simulink model "lead_increasing_space_gap"  (R2025a)
settings: Solver=VariableStepAuto  StartTime=0.0  StopTime=20  RelTol=1e-3
settings Model: Creator=sanborkl  LastModifiedBy=sanborkl

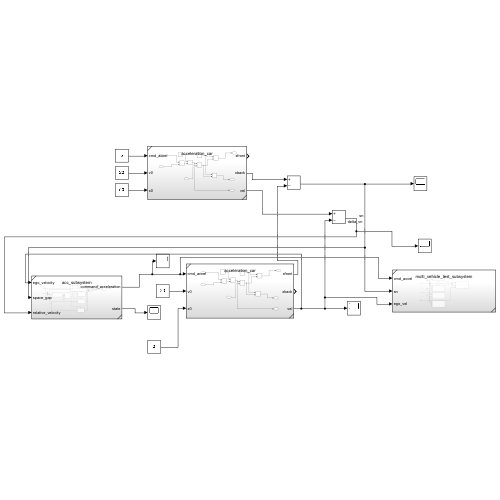
[thumbnail: Simulink's stored preview of the top-level diagram]
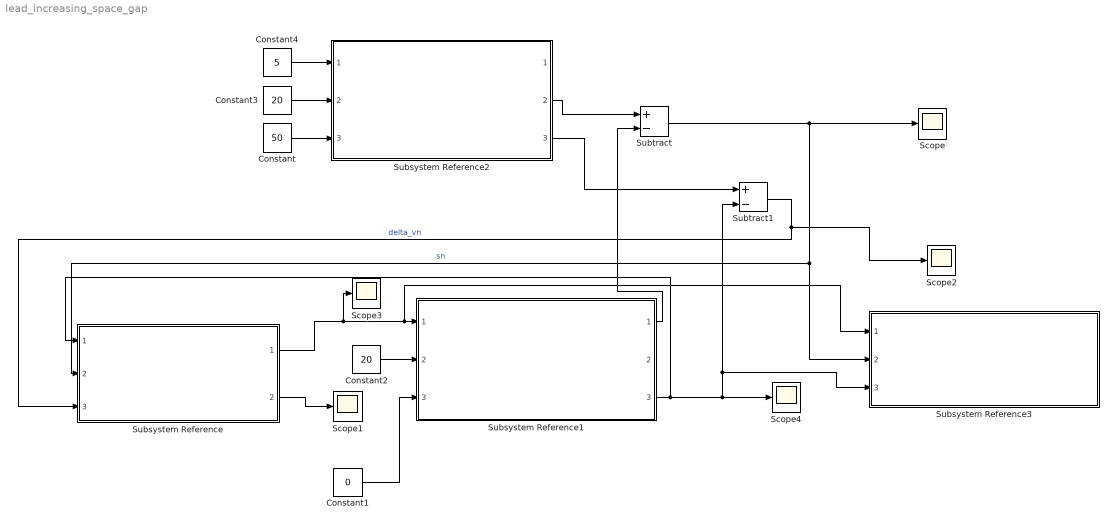
== system lead_increasing_space_gap ==
  Constant : Constant  Value=50
  Constant1 : Constant  Value=0
  Constant2 : Constant  Value=20
  Constant3 : Constant  Value=20
  Constant4 : Constant  Value=5
  Scope{,1..4} (5 alike) : Scope
      Scope settings: ActiveDisplayYMinimum=7.0577298305674168  ActiveDisplayYMaximum=50.060252241048069
      Scope1 settings: ActiveDisplayYMinimum=-1  ActiveDisplayYMaximum=1  DataLoggingVariableName=ScopeData2
      Scope2 settings: ActiveDisplayYMinimum=-1  ActiveDisplayYMaximum=1  DataLoggingVariableName=ScopeData3
      Scope3 settings: ActiveDisplayYMinimum=0.5  ActiveDisplayYMaximum=2.5  DataLoggingVariableName=ScopeData4
      Scope4 settings: ActiveDisplayYMinimum=16.249999999999993  ActiveDisplayYMaximum=53.750000000000078
  Subsystem Reference : Subsystem  ReferencedSubsystem=acc_subsystem
  Subsystem Reference1 : Subsystem  ReferencedSubsystem=acceleration_car
  Subsystem Reference2 : Subsystem  ReferencedSubsystem=acceleration_car
  Subsystem Reference3 : Subsystem  ReferencedSubsystem=multi_vehicle_test_subsystem
  Subtract : Sum  Inputs=+-
  Subtract1 : Sum  Inputs=+-
  wires:
  Subsystem Reference2/3 -> Subtract1/1
  Constant3/1 -> Subsystem Reference2/2
  Constant/1 -> Subsystem Reference2/3
  Constant2/1 -> Subsystem Reference1/2
  Subsystem Reference1/1 -> Subtract/2
  Subsystem Reference/1 -> Scope3/1, Subsystem Reference3/1, Subsystem Reference1/1
  Constant1/1 -> Subsystem Reference1/3
  Subsystem Reference/2 -> Scope1/1
  Subsystem Reference2/2 -> Subtract/1
  Subtract/1 -> Subsystem Reference3/2, Subsystem Reference/2, Scope/1  "sn"
  Subsystem Reference1/3 -> Subsystem Reference/1, Subtract1/2, Subsystem Reference3/3, Scope4/1
  Subtract1/1 -> Scope2/1, Subsystem Reference/3  "delta_vn"
  Constant4/1 -> Subsystem Reference2/1
